simulink subsystem "s0518_swing_up_controller2"  (R2019b)
settings: Solver=VariableStepAuto  StartTime=0.0  StopTime=10.0  RelTol=1e-3
undefined symbols (not defined in the file): __PRM__SERIALIZED__DATA__, den_ref_filter, DiscIntNeverNeededParam, dt_control, num_ref_filter, PARAMS, SubsystemReferenceBlock
libraries: simulink x5
settings Model: Creator=paolo  LastModifiedBy=giaco

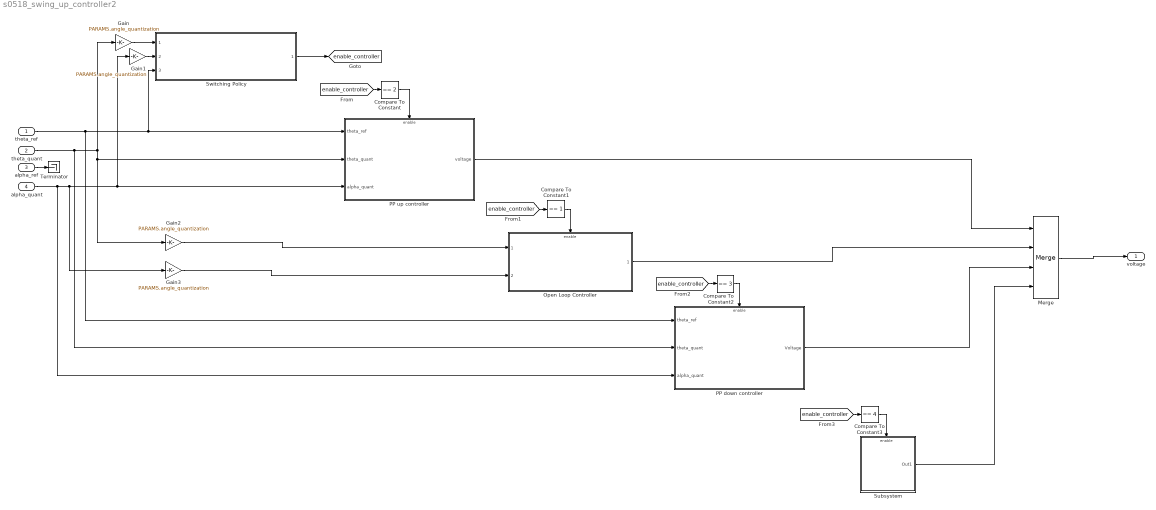
== system s0518_swing_up_controller2 ==
  theta_ref : Inport
  theta_quant : Inport  Port=2
  alpha_ref : Inport  Port=3
  alpha_quant : Inport  Port=4
  Compare To Constant : simulink/Logic and Bit Operations/Compare To Constant  relop===  const=2  OutDataTypeStr=boolean
  Compare To Constant1 : simulink/Logic and Bit Operations/Compare To Constant  relop===  const=1  OutDataTypeStr=boolean
  Compare To Constant2 : simulink/Logic and Bit Operations/Compare To Constant  relop===  const=3  OutDataTypeStr=boolean
  Compare To Constant3 : simulink/Logic and Bit Operations/Compare To Constant  relop===  const=4  OutDataTypeStr=boolean
  Gain{,1..3} (4 alike) : Gain  Gain=PARAMS.angle_quantization
  Merge : Merge  Inputs=4
  Open Loop Controller : Subsystem  BlockKeywords=__PRM__SERIALIZED__DATA__:SubsystemReferenceBlock  ReferencedSubsystem=s0519_Better_Lyapunov_maybe  k_E=1  k_th=PARAMS.k_th  k_delta=PARAMS.k_delta  k_ome=PARAMS.k_ome
  PP down controller : Subsystem
  PP up controller : Subsystem
  Subsystem : Subsystem
  Switching Policy : Subsystem  BlockKeywords=__PRM__SERIALIZED__DATA__:SubsystemReferenceBlock  ReferencedSubsystem=s0518_switching_policy3
  Terminator : Terminator
  voltage : Outport
  tag scope: enable_controller=global
  wires:
  alpha_quant/1 -> Gain3/1, PP up controller/3(alpha_quant), Gain1/1, PP down controller/3(alpha_quant)
  Merge/1 -> voltage/1
  alpha_ref/1 -> Terminator/1
  theta_quant/1 -> Gain2/1, PP up controller/2(theta_quant), Gain/1, PP down controller/2(theta_quant)
  theta_ref/1 -> PP up controller/1(theta_ref), Switching Policy/3, PP down controller/1(theta_ref)
  PP up controller/1(voltage) -> Merge/1
  Switching Policy/1 -> [enable_controller]
  Gain/1 -> Switching Policy/1
  Gain1/1 -> Switching Policy/2
  Gain2/1 -> Open Loop Controller/1
  Gain3/1 -> Open Loop Controller/2
  Open Loop Controller/1 -> Merge/2
  PP down controller/1(Voltage) -> Merge/3
  [enable_controller] -> Compare To Constant/1
  Compare To Constant/1 -> PP up controller/Enable
  [enable_controller] -> Compare To Constant1/1
  Compare To Constant2/1 -> PP down controller/Enable
  [enable_controller] -> Compare To Constant2/1
  Compare To Constant1/1 -> Open Loop Controller/Enable
  Compare To Constant3/1 -> Subsystem/Enable
  [enable_controller] -> Compare To Constant3/1
  Subsystem/1(Out1) -> Merge/4

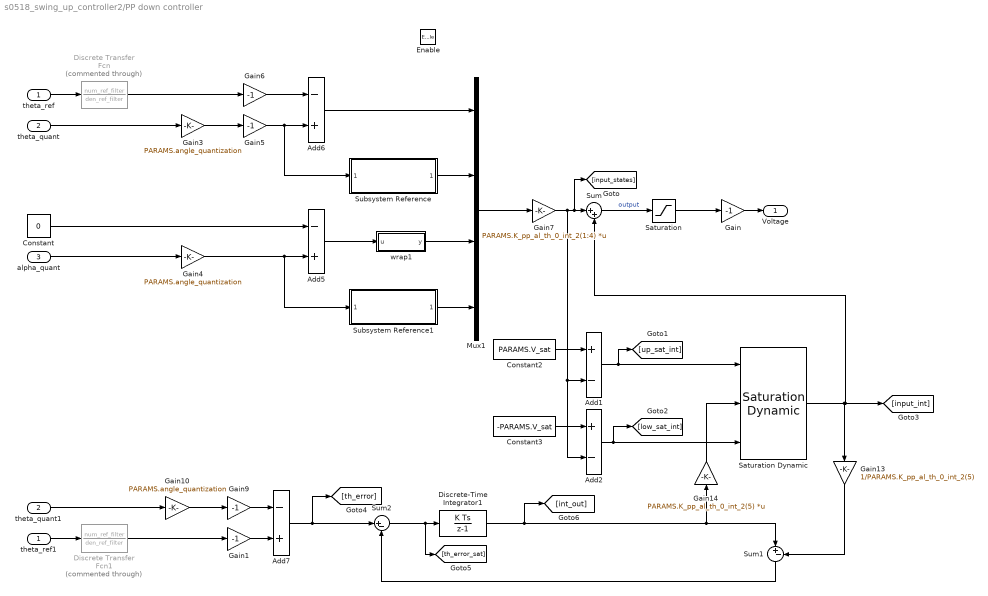
== system s0518_swing_up_controller2/PP down controller ==
  theta_ref : Inport
  theta_quant : Inport  Port=2
  alpha_quant : Inport  Port=3
  Enable : EnablePort  StatesWhenEnabling=reset
  Add1 : Sum  Inputs=+-
  Add2 : Sum  Inputs=+-
  Add5 : Sum  Inputs=-+
  Add6 : Sum  Inputs=-+
  Add7 : Sum  Inputs=-+
  Constant : Constant  Value=0
  Constant2 : Constant  Value=PARAMS.V_sat
  Constant3 : Constant  Value=-PARAMS.V_sat
  Discrete Transfer Fcn : DiscreteTransferFcn  Commented=through  Numerator=num_ref_filter  Denominator=den_ref_filter
  Discrete Transfer Fcn1 : DiscreteTransferFcn  Commented=through  Numerator=num_ref_filter  Denominator=den_ref_filter
  Discrete-Time Integrator1 : DiscreteIntegrator  SampleTime=-1  ICPrevOutput=DiscIntNeverNeededParam  ICPrevScaledInput=DiscIntNeverNeededParam
  Gain{,1,5..6,9} (5 alike) : Gain  Gain=-1
  Gain10 : Gain  Gain=PARAMS.angle_quantization
  Gain13 : Gain  Gain=1/PARAMS.K_pp_al_th_0_int_2(5)
  Gain14 : Gain  Gain=PARAMS.K_pp_al_th_0_int_2(5)  Multiplication=Matrix(K*u)
  Gain3 : Gain  Gain=PARAMS.angle_quantization
  Gain4 : Gain  Gain=PARAMS.angle_quantization
  Gain7 : Gain  Gain=PARAMS.K_pp_al_th_0_int_2(1:4)  Multiplication=Matrix(K*u)
  Mux1 : Mux
  Saturation : Saturate  UpperLimit=PARAMS.V_sat  LowerLimit=-PARAMS.V_sat
  Saturation Dynamic : simulink/Discontinuities/Saturation Dynamic  OutMin=[]  OutMax=[]  OutDataTypeStr=Inherit: Same as second input  OutDataType=fixdt(1, 16)  OutScaling=2^-10  DoSatur=off
  Subsystem Reference : Subsystem  BlockKeywords=__PRM__SERIALIZED__DATA__:SubsystemReferenceBlock  ReferencedSubsystem=Filtered_Derivative  num=num_der_filter  den=den_der_filter
  Subsystem Reference1 : Subsystem  BlockKeywords=__PRM__SERIALIZED__DATA__:SubsystemReferenceBlock  ReferencedSubsystem=Filtered_Derivative  num=num_der_filter  den=den_der_filter
  Sum : Sum  Inputs=|++
  Sum1 : Sum  Inputs=|+-
  Sum2 : Sum  Inputs=|+-
  theta_quant1 : InportShadow  Port=2
  theta_ref1 : InportShadow
  wrap1 : MATLAB Function  TreatAsAtomicUnit=on
  Voltage : Outport
  wires:
  Subsystem Reference1/1 -> Mux1/4
  Gain5/1 -> Add6/2, Subsystem Reference/1
  Constant/1 -> Add5/1
  Gain6/1 -> Add6/1
  Discrete-Time Integrator1/1 -> Gain14/1, Sum1/1, [int_out]
  Saturation/1 -> Gain/1
  Sum/1 -> Saturation/1  "output"
  theta_ref1/1 -> Discrete Transfer Fcn1/1
  theta_quant1/1 -> Gain10/1
  Gain1/1 -> Add7/2
  Discrete Transfer Fcn1/1 -> Gain1/1
  alpha_quant/1 -> Gain4/1
  theta_quant/1 -> Gain3/1
  Gain9/1 -> Add7/1
  Gain/1 -> Voltage/1
  Gain3/1 -> Gain5/1
  Add1/1 -> Saturation Dynamic/1, [up_sat_int]
  Add2/1 -> Saturation Dynamic/3, [low_sat_int]
  Discrete Transfer Fcn/1 -> Gain6/1
  Saturation Dynamic/1 -> Gain13/1, [input_int], Sum/2
  Gain4/1 -> Add5/2, Subsystem Reference1/1
  Constant2/1 -> Add1/1
  Sum1/1 -> Sum2/2
  wrap1/1(y) -> Mux1/3
  Add7/1 -> [th_error], Sum2/1
  Subsystem Reference/1 -> Mux1/2
  Constant3/1 -> Add2/1
  Add5/1 -> wrap1/1(u)
  Gain10/1 -> Gain9/1
  Mux1/1 -> Gain7/1
  Sum2/1 -> Discrete-Time Integrator1/1, [th_error_sat]
  Gain13/1 -> Sum1/2
  Add6/1 -> Mux1/1
  theta_ref/1 -> Discrete Transfer Fcn/1
  Gain7/1 -> Sum/1, [input_states], Add2/2, Add1/2
  Gain14/1 -> Saturation Dynamic/2

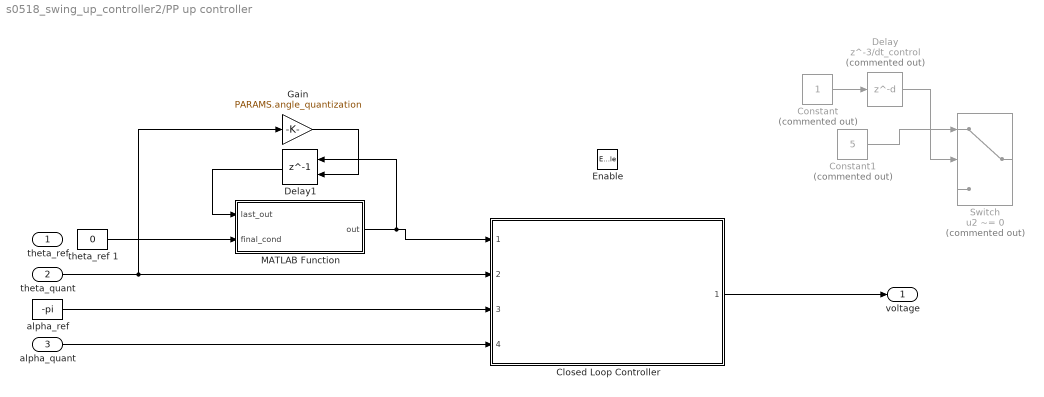
== system s0518_swing_up_controller2/PP up controller ==
  theta_ref : Inport
  theta_quant : Inport  Port=2
  alpha_quant : Inport  Port=3
  Enable : EnablePort  StatesWhenEnabling=reset
  Closed Loop Controller : Subsystem  BlockKeywords=__PRM__SERIALIZED__DATA__:SubsystemReferenceBlock  ReferencedSubsystem=s0320_alpha_theta_PP
  Constant : Constant  Commented=on
  Constant1 : Constant  Commented=on  Value=5
  Delay : Delay  Commented=on  DelayLength=3/dt_control
  Delay1 : Delay  DelayLength=1  InitialConditionSource=Input port
      settings: InputPortMap=u0,p4
  Gain : Gain  Gain=PARAMS.angle_quantization
  MATLAB Function : MATLAB Function  TreatAsAtomicUnit=on
  Switch : Switch  Commented=on  Criteria=u2 ~= 0
  "alpha_ref " : Constant  Value=-pi
  theta_ref 1 : Constant  Value=0
  voltage : Outport
  wires:
  theta_ref 1/1 -> MATLAB Function/2(final_cond)
  Constant1/1 -> Switch/1
  Constant/1 -> Delay/1
  Delay/1 -> Switch/2
  Delay1/1 -> MATLAB Function/1(last_out)
  Gain/1 -> Delay1/2
  MATLAB Function/1(out) -> Closed Loop Controller/1, Delay1/1
  Closed Loop Controller/1 -> voltage/1
  "alpha_ref "/1 -> Closed Loop Controller/3
  alpha_quant/1 -> Closed Loop Controller/4
  theta_quant/1 -> Gain/1, Closed Loop Controller/2

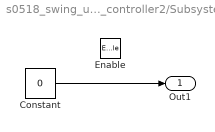
== system s0518_swing_up_controller2/Subsystem ==
  Enable : EnablePort  StatesWhenEnabling=reset
  Constant : Constant  Value=0
  Out1 : Outport
  wires:
  Constant/1 -> Out1/1

== matlab function s0518_swing_up_controller2/PP down controller/wrap1 ==
  data: u input; y output
function y = wrap(u)
stop_condition = false;
y = u;
while ~stop_condition
    if y > pi
        y = y - 2*pi;
    elseif y < -pi
        y = y + 2*pi;
    else
        stop_condition = true;
    end
end

== matlab function s0518_swing_up_controller2/PP up controller/MATLAB Function ==
  data: last_out input; out output; final_cond input; dt_control parameter
function out = fcn(last_out, final_cond, dt_control)

out = last_out + (final_cond - last_out)/0.2*dt_control;
